simulink model "Ball_Plate_Simulation"  (R2018a)
settings: Solver=VariableStepAuto  StartTime=0.0  StopTime=30  RelTol=1e-3
values from neighbouring files (symbols this model uses):
  A = [ 0 1 0 0; 0 (-5/7)*(fc/mb) (+5/7)*g 0; 0 0 0 1; 0 0 -(Wn^2) -2*Eta*Wn]    [State_space.m]    (also in matlab.mat = [0 0 0 0 1 -0.310559006211 0 0 0 7.00714285714 0 -357.777225)
  A2 = [ 0 1 0 0; 0 (-5/7)*(fc/mb) (+5/7)*g 0; 0 0 0 1; 0 0 -(Wn^2) -2*Eta*Wn]    [State_space.m]    (also in matlab.mat = [0 0 0 0 1 -0.310559006211 0 0 0 7.00714285714 0 -357.777225)
  B = [ 0 ; 0 ; 0 ; Wn^2]    [State_space.m]    (also in matlab.mat = [0 0 0 357.777225])
  B2 = [ 0 ; 0 ; 0 ; Wn^2]    [State_space.m]    (also in matlab.mat = [0 0 0 357.777225])
  C = [ 1 0 0 0]    [State_space.m]    (also in matlab.mat = [1 0 0 0])
  C2 = [ 1 0 0 0; 0 0 1 0; 0 0 K 0; 0 0 0 0]    [State_space.m]    (also in matlab.mat = [1 0 0 0 0 0 0 0 0 1 3.64705882353 0 ... (16 elements, 4x4)])
  D = zeros(1,1)    [State_space.m]    (also in matlab.mat = 0)
  D2 = [ 0 ; 0 ; 0; K]    [State_space.m]    (also in matlab.mat = [0 0 0 3.64705882353])
  Eta = 1.0087    [State_space.m]    (also in matlab.mat)
  fc = 0.02    [State_space.m]    (also in matlab.mat)
  g = 9.81    [State_space.m]    (also in matlab.mat)
  mb = 0.046    [State_space.m]    (also in matlab.mat)
  Wn = 18.915    [State_space.m]    (also in matlab.mat)
libraries: simulink x3
settings Model: Creator=JISA  LastModifiedBy=JISA

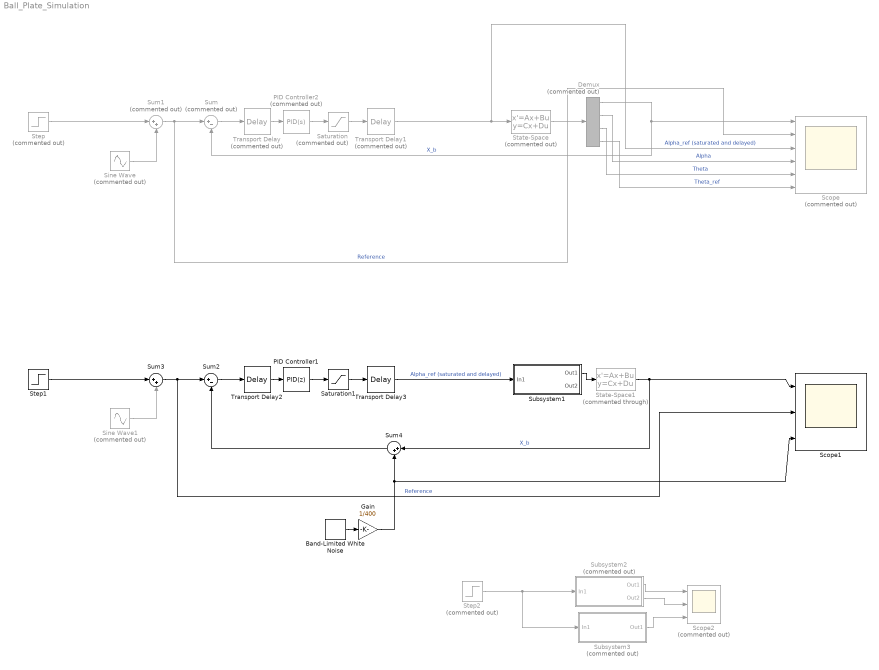
== system Ball_Plate_Simulation ==
  Band-Limited White Noise : simulink/Sources/Band-Limited White Noise  Cov=[0.01]  Ts=0.01  seed=[23341]
  Demux : Demux  Commented=on
  Gain : Gain  Gain=1/400
  PID Controller1 : simulink/Continuous/PID Controller  Controller=PID  TimeDomain=Discrete-time  SampleTime=-1  IntegratorMethod=Forward Euler  FilterMethod=Backward Euler  Form=Parallel  UseFilter=on  ControllerParametersSource=internal  P=0.0444682512900468  I=0.00285212339320274  D=0.168273746466015  N=131.614475836593  InitialConditionSource=internal  InitialConditionForIntegrator=0  InitialConditionForFilter=0  ExternalReset=none  LimitOutput=off  UpperSaturationLimit=inf  LowerSaturationLimit=-inf  LinearizeAsGain=on  AntiWindupMode=none  Kb=1  TrackingMode=off  Kt=1  PParamMin=[]  PParamMax=[]  IParamMin=[]  IParamMax=[]  DParamMin=[]  DParamMax=[]  NParamMin=[]  NParamMax=[]  KbParamMin=[]  KbParamMax=[]  KtParamMin=[]  KtParamMax=[]  POutMin=[]  POutMax=[]  IOutMin=[]  IOutMax=[]  DOutMin=[]  DOutMax=[]  NOutMin=[]  NOutMax=[]  KbOutMin=[]  KbOutMax=[]  KtOutMin=[]  KtOutMax=[]  IntegratorOutMin=[]  IntegratorOutMax=[]  FilterOutMin=[]  FilterOutMax=[]  SumOutMin=[]  SumOutMax=[]  SumI1OutMin=[]  SumI1OutMax=[]  SumI2OutMin=[]  SumI2OutMax=[]  SumI3OutMin=[]  SumI3OutMax=[]  SumDOutMin=[]  SumDOutMax=[]  SaturationOutMin=[]  SaturationOutMax=[]  IntegratorContinuousStateAttributes=''  IntegratorStateMustResolveToSignalObject=off  IntegratorRTWStateStorageClass=Auto  FilterContinuousStateAttributes=''  FilterStateMustResolveToSignalObject=off  FilterRTWStateStorageClass=Auto  DifferentiatorICPrevScaledInput=0  DifferentiatorOutMin=[]  DifferentiatorOutMax=[]  FilterDiffOutCoefMin=[]  FilterDiffOutCoefMax=[]  SumDenOutMin=[]  SumDenOutMax=[]  SumNumOutMin=[]  SumNumOutMax=[]  ReciprocalOutMin=[]  ReciprocalOutMax=[]  DivideOutMin=[]  DivideOutMax=[]  TunerSelectOption=Transfer Function Based (PID Tuner App)
  PID Controller2 : simulink/Continuous/PID Controller  Commented=on  Controller=PID  TimeDomain=Continuous-time  SampleTime=-1  IntegratorMethod=Forward Euler  FilterMethod=Forward Euler  Form=Parallel  UseFilter=on  ControllerParametersSource=internal  P=0.0513289639999758  I=0.000338203351989916  D=0.0796060238531818  N=1.6153069625007  InitialConditionSource=internal  InitialConditionForIntegrator=0  InitialConditionForFilter=0  ExternalReset=none  LimitOutput=off  UpperSaturationLimit=inf  LowerSaturationLimit=-inf  LinearizeAsGain=on  AntiWindupMode=none  Kb=1  TrackingMode=off  Kt=1  PParamMin=[]  PParamMax=[]  IParamMin=[]  IParamMax=[]  DParamMin=[]  DParamMax=[]  NParamMin=[]  NParamMax=[]  KbParamMin=[]  KbParamMax=[]  KtParamMin=[]  KtParamMax=[]  POutMin=[]  POutMax=[]  IOutMin=[]  IOutMax=[]  DOutMin=[]  DOutMax=[]  NOutMin=[]  NOutMax=[]  KbOutMin=[]  KbOutMax=[]  KtOutMin=[]  KtOutMax=[]  IntegratorOutMin=[]  IntegratorOutMax=[]  FilterOutMin=[]  FilterOutMax=[]  SumOutMin=[]  SumOutMax=[]  SumI1OutMin=[]  SumI1OutMax=[]  SumI2OutMin=[]  SumI2OutMax=[]  SumI3OutMin=[]  SumI3OutMax=[]  SumDOutMin=[]  SumDOutMax=[]  SaturationOutMin=[]  SaturationOutMax=[]  IntegratorContinuousStateAttributes=''  IntegratorStateMustResolveToSignalObject=off  IntegratorRTWStateStorageClass=Auto  FilterContinuousStateAttributes=''  FilterStateMustResolveToSignalObject=off  FilterRTWStateStorageClass=Auto  DifferentiatorICPrevScaledInput=0  DifferentiatorOutMin=[]  DifferentiatorOutMax=[]  FilterDiffOutCoefMin=[]  FilterDiffOutCoefMax=[]  SumDenOutMin=[]  SumDenOutMax=[]  SumNumOutMin=[]  SumNumOutMax=[]  ReciprocalOutMin=[]  ReciprocalOutMax=[]  DivideOutMin=[]  DivideOutMax=[]  TunerSelectOption=Transfer Function Based (PID Tuner App)
  Saturation : Saturate  Commented=on  UpperLimit=15  LowerLimit=-15
  Saturation1 : Saturate  UpperLimit=15  LowerLimit=-15
  Scope : Scope  Commented=on  NumInputPorts=6
  Scope1 : Scope  NumInputPorts=3
  Scope2 : Scope  Commented=on  NumInputPorts=3
  Sine Wave : Sin  Commented=on  Amplitude=5  SampleTime=0
  Sine Wave1 : Sin  Commented=on  Amplitude=5  SampleTime=0
  State-Space : StateSpace  Commented=on  A=A2  B=B2  C=C2  D=D2  InitialCondition=0
  State-Space1 : StateSpace  Commented=through  A=A  B=B  C=C  D=D  InitialCondition=0
  Step : Step  Commented=on  Time=0  SampleTime=0
  Step1 : Step  Time=0  After=0.1  SampleTime=0
  Step2 : Step  Commented=on  Time=0  After=15  SampleTime=0
  Subsystem1 : Subsystem
  Subsystem2 : Subsystem  Commented=on
  Subsystem3 : Subsystem  Commented=on
  Sum : Sum  Commented=on  Inputs=|+-
  Sum1 : Sum  Commented=on  Inputs=|++
  Sum2 : Sum  Inputs=|+-
  Sum3 : Sum  Inputs=|++
  Sum4 : Sum  Inputs=|++
  Transport Delay : TransportDelay  Commented=on  DelayTime=0.2
  Transport Delay1 : TransportDelay  Commented=on  DelayTime=0.05
  Transport Delay2 : TransportDelay  DelayTime=0.2
  Transport Delay3 : TransportDelay  DelayTime=0.05
  wires:
  PID Controller2/1 -> Saturation/1
  Sum/1 -> Transport Delay/1
  Transport Delay/1 -> PID Controller2/1
  Saturation/1 -> Transport Delay1/1
  Step/1 -> Sum1/1
  Sine Wave/1 -> Sum1/2
  Sum1/1 -> Scope/2, Sum/1  "Reference"
  State-Space/1 -> Demux/1
  Demux/1 -> Sum/2, Scope/1  "X_b"
  Demux/2 -> Scope/4  "Alpha"
  Demux/3 -> Scope/5  "Theta"
  Demux/4 -> Scope/6  "Theta_ref"
  Transport Delay1/1 -> Scope/3, State-Space/1  "Alpha_ref (saturated and delayed)"
  Sine Wave1/1 -> Sum3/2
  Transport Delay3/1 -> Subsystem1/1(In1)  "Alpha_ref (saturated and delayed)"
  State-Space1/1 -> Sum4/1, Scope1/1  "X_b"
  Sum3/1 -> Scope1/2, Sum2/1  "Reference"
  Saturation1/1 -> Transport Delay3/1
  Transport Delay2/1 -> PID Controller1/1
  Sum2/1 -> Transport Delay2/1
  PID Controller1/1 -> Saturation1/1
  Step1/1 -> Sum3/1
  Step2/1 -> Subsystem3/1(In1), Subsystem2/1(In1)
  Subsystem1/1(Out1) -> State-Space1/1
  Subsystem3/1(Out1) -> Scope2/3
  Subsystem2/1(Out1) -> Scope2/1
  Subsystem2/2(Out2) -> Scope2/2
  Sum4/1 -> Sum2/2
  Band-Limited White Noise/1 -> Gain/1
  Gain/1 -> Scope1/3, Sum4/2

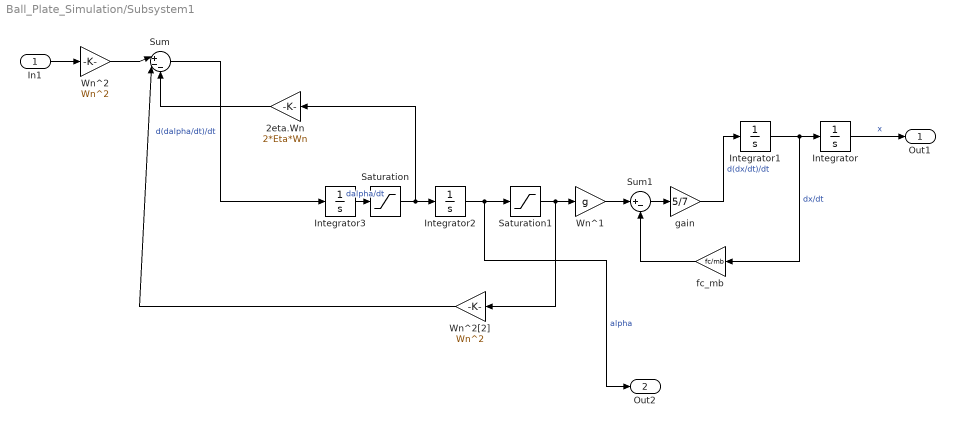
== system Ball_Plate_Simulation/Subsystem1 ==
  In1 : Inport
  2eta.Wn : Gain  Gain=2*Eta*Wn
  Integrator{,1..3} (4 alike) : Integrator
  Saturation : Saturate  UpperLimit=33.9341  LowerLimit=-33.9341
  Saturation1 : Saturate  UpperLimit=14.5  LowerLimit=-14.5
  Sum : Sum  Inputs=|+--
  Sum1 : Sum  Inputs=|+-
  Wn^1 : Gain  Gain=g
  Wn^2 : Gain  Gain=Wn^2
  Wn^2[2] : Gain  Gain=Wn^2
  fc_mb : Gain  Gain=fc/mb
  gain : Gain  Gain=5/7
  Out1 : Outport
  Out2 : Outport  Port=2
  wires:
  In1/1 -> Wn^2/1
  Wn^2/1 -> Sum/1
  Integrator/1 -> Out1/1  "x"
  Integrator1/1 -> fc_mb/1, Integrator/1  "dx/dt"
  gain/1 -> Integrator1/1  "d(dx/dt)/dt"
  Integrator2/1 -> Out2/1, Saturation1/1  "alpha"
  Wn^1/1 -> Sum1/1
  fc_mb/1 -> Sum1/2
  Sum1/1 -> gain/1
  Sum/1 -> Integrator3/1  "d(dalpha/dt)/dt"
  Wn^2[2]/1 -> Sum/2
  2eta.Wn/1 -> Sum/3
  Saturation/1 -> 2eta.Wn/1, Integrator2/1
  Integrator3/1 -> Saturation/1  "dalpha/dt"
  Saturation1/1 -> Wn^2[2]/1, Wn^1/1

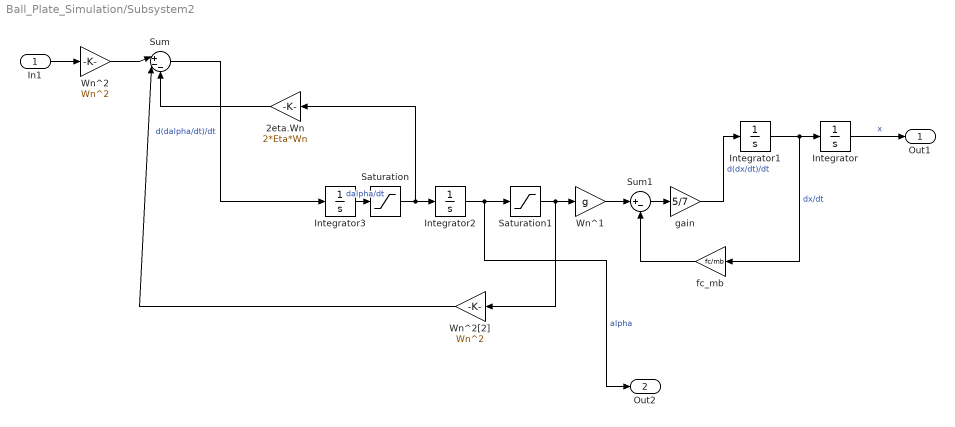
== system Ball_Plate_Simulation/Subsystem2 ==
  In1 : Inport
  2eta.Wn : Gain  Gain=2*Eta*Wn
  Integrator{,1..3} (4 alike) : Integrator
  Saturation : Saturate  UpperLimit=97.58  LowerLimit=-97.58
  Saturation1 : Saturate  UpperLimit=14.5  LowerLimit=-14.5
  Sum : Sum  Inputs=|+--
  Sum1 : Sum  Inputs=|+-
  Wn^1 : Gain  Gain=g
  Wn^2 : Gain  Gain=Wn^2
  Wn^2[2] : Gain  Gain=Wn^2
  fc_mb : Gain  Gain=fc/mb
  gain : Gain  Gain=5/7
  Out1 : Outport
  Out2 : Outport  Port=2
  wires:
  In1/1 -> Wn^2/1
  Wn^2/1 -> Sum/1
  Integrator/1 -> Out1/1  "x"
  Integrator1/1 -> fc_mb/1, Integrator/1  "dx/dt"
  gain/1 -> Integrator1/1  "d(dx/dt)/dt"
  Integrator2/1 -> Out2/1, Saturation1/1  "alpha"
  Wn^1/1 -> Sum1/1
  fc_mb/1 -> Sum1/2
  Sum1/1 -> gain/1
  Sum/1 -> Integrator3/1  "d(dalpha/dt)/dt"
  Wn^2[2]/1 -> Sum/2
  2eta.Wn/1 -> Sum/3
  Saturation/1 -> 2eta.Wn/1, Integrator2/1
  Integrator3/1 -> Saturation/1  "dalpha/dt"
  Saturation1/1 -> Wn^2[2]/1, Wn^1/1

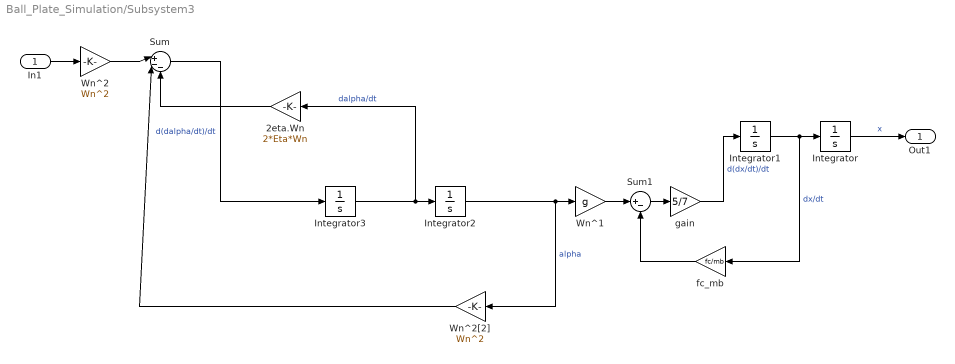
== system Ball_Plate_Simulation/Subsystem3 ==
  In1 : Inport
  2eta.Wn : Gain  Gain=2*Eta*Wn
  Integrator{,1..3} (4 alike) : Integrator
  Sum : Sum  Inputs=|+--
  Sum1 : Sum  Inputs=|+-
  Wn^1 : Gain  Gain=g
  Wn^2 : Gain  Gain=Wn^2
  Wn^2[2] : Gain  Gain=Wn^2
  fc_mb : Gain  Gain=fc/mb
  gain : Gain  Gain=5/7
  Out1 : Outport
  wires:
  In1/1 -> Wn^2/1
  Wn^2/1 -> Sum/1
  Integrator/1 -> Out1/1  "x"
  Integrator1/1 -> fc_mb/1, Integrator/1  "dx/dt"
  gain/1 -> Integrator1/1  "d(dx/dt)/dt"
  Integrator2/1 -> Wn^2[2]/1, Wn^1/1  "alpha"
  Wn^1/1 -> Sum1/1
  fc_mb/1 -> Sum1/2
  Sum1/1 -> gain/1
  Sum/1 -> Integrator3/1  "d(dalpha/dt)/dt"
  Wn^2[2]/1 -> Sum/2
  2eta.Wn/1 -> Sum/3
  Integrator3/1 -> 2eta.Wn/1, Integrator2/1  "dalpha/dt"
